simulink model "MotorsFlatSpeed"  (R2019a)
settings: Solver=FixedStepAuto  StartTime=0.0  StopTime=2.0  FixedStep=Ts  RelTol=1e-3  EnableMultiTasking=on
InitFcn:
  | run('../model.m')
libraries: legoev3lib x4
settings Model: SimulationMode=external  ExtModeTrigDuration=2  Creator=thh206  LastModifiedBy=thh206
settings SolverCC: PositivePriorityOrder=on
settings DataIOCC: ReturnWorkspaceOutputs=off
settings OptimizationCC: EnhancedBackFolding=on  PassReuseOutputArgsAs=Individual arguments  MaxStackSize=64  OptimizeBlockOrder=speed  DifferentSizesBufferReuse=on  OptimizationCustomize=off
settings DebuggingCC: ParameterTunabilityLossMsg=error  PregeneratedLibrarySubsystemCodeDiagnostic=none  ArithmeticOperatorsInVariantConditions=warning
settings HardwareCC: ProdBitPerPointer=32  ProdBitPerSizeT=32  ProdBitPerPtrDiffT=32  ProdLargestAtomicInteger=Long  ProdWordSize=32  ProdHWDeviceType=ARM Compatible->ARM 9
settings SFSimCC: SimUseLocalCustomCode=off  MATLABDynamicMemAlloc=off
settings RTWCC: SystemTargetFile=ert.tlc  HardwareBoard=LEGO MINDSTORMS EV3  TLCOptions="-aInlineSetEventsForThisBaseRateFcn=TLC_FALSE -aSuppressMultiTaskScheduler=TLC_FALSE  -aRateBasedStepFcn=0"  TemplateMakefile=ert_default_tmf  GenerateReport=on  RTWUseLocalCustomCode=off  Toolchain=Sourcery G++ Lite v2009q3  IncludeHyperlinkInReport=on  LaunchReport=on  GenerateTraceInfo=on  GenerateTraceReport=on  GenerateTraceReportSl=on  GenerateTraceReportSf=on  GenerateTraceReportEml=on
settings CodeAppCC: ForceParamTrailComments=on  IgnoreCustomStorageClasses=off  OperatorAnnotations=on  SimulinkDataObjDesc=on  SFDataObjDesc=on  InsertBlockDesc=on
settings ERTTargetCC: SupportContinuousTime=on  SupportVariableSizeSignals=on

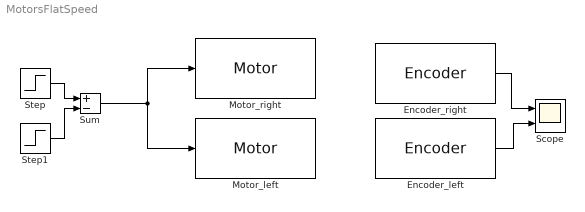
== system MotorsFlatSpeed ==
  Encoder_left : legoev3lib/Encoder  portNumber=D  opMode=No reset  sampleTime=Ts
      settings: SourceProductName=Simulink Support Package for LEGO MINDSTORMS EV3 Hardware  SourceProductBaseCode=LEGOEV3
  Encoder_right : legoev3lib/Encoder  portNumber=A  opMode=No reset  sampleTime=Ts
      settings: SourceProductName=Simulink Support Package for LEGO MINDSTORMS EV3 Hardware  SourceProductBaseCode=LEGOEV3
  Motor_left : legoev3lib/Motor  sportNumber=D  sstopAction=Brake
  Motor_right : legoev3lib/Motor  sportNumber=A  sstopAction=Brake
  Scope : Scope  NumInputPorts=2
  Step : Step  After=100  SampleTime=0
  Step1 : Step  Time=2.0  After=100  SampleTime=0
  Sum : Sum  Inputs=+-
  wires:
  Encoder_left/1 -> Scope/2
  Sum/1 -> Motor_left/1, Motor_right/1
  Encoder_right/1 -> Scope/1
  Step/1 -> Sum/1
  Step1/1 -> Sum/2
